simulink model "UAV_HIL"  (Simulink 8.0)
settings: Solver=ode3  StartTime=0.0  StopTime=inf  FixedStep=SampleTime  RelTol=1e-3
values from neighbouring files (symbols this model uses):
  SampleTime = 0.01    [setup.m]
undefined symbols (not defined in the file or in its folder): Serial_Port, Standard_Devices
undefined symbols (not defined in the file): AC
libraries: Actuator_Lib x2, rtwinlib x2, Environment_Lib x1, simulink x1, NonlinearModel_Lib x1, Sensors_Lib x1
CloseFcn:
  | rtwprivate ssgencode ModelCloseRequest Good_NL_model
settings Model: Creator=Paul  LastModifiedBy=brtaylor  SimulationMode=external  ExtModeTrigDuration=100000
settings DataIOCC: SignalLoggingSaveFormat=ModelDataLogs  TimeSaveName=time
settings OptimizationCC: InitFltsAndDblsToZero=on
settings DebuggingCC: ParameterPrecisionLossMsg=none  FcnCallInpInsideContextMsg=UseLocalSettings  StrictBusMsg=Warning
settings HardwareCC: ProdIntDivRoundTo=Zero  ProdEndianess=LittleEndian  ProdHWDeviceType=Generic->32-bit x86 compatible
settings SFSimCC: SimParseCustomCode=off
settings RTWCC: SystemTargetFile=rtwin.tlc  TemplateMakefile=rtwin.tmf  Description=Real-Time Windows Target  ProcessScript=rtwin_make_rtw_hook  RTWCompilerOptimization=On
settings CodeAppCC: MaxIdLength=95
settings RTWinTargetCC: TargetLibSuffix=_rtwin.lib  TargetPreCompLibLocation=C:\Program Files\MATLAB\R2012b\toolbox\rtw\targets\rtwin\lib\win64  CodeReplacementLibrary=ANSI_C  RTWinDir=C:/PROGRA~1/MATLAB/R2012b/toolbox/rtw/targets/rtwin  TargetArch=win64

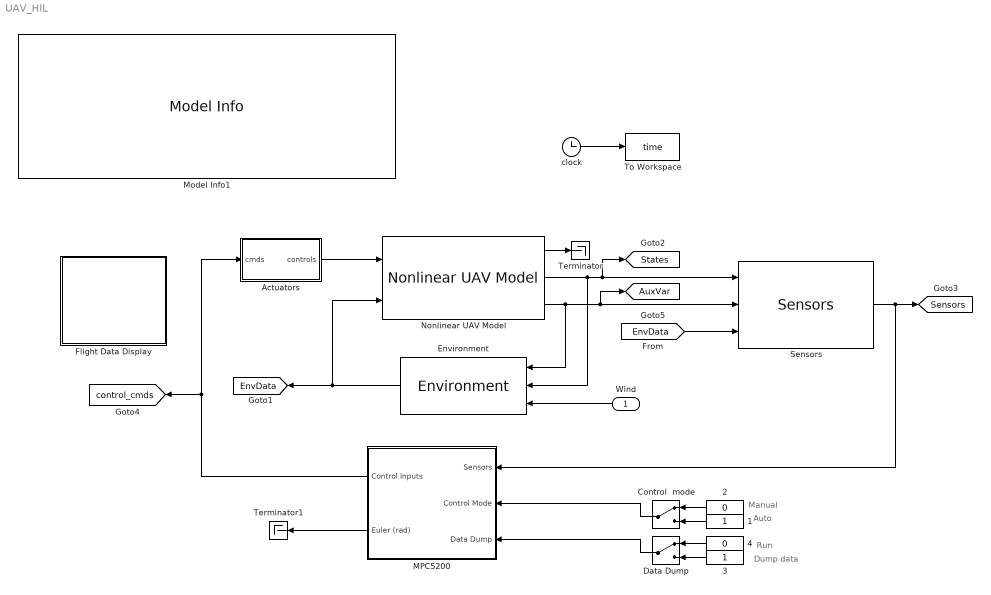
== system UAV_HIL ==
  note: Auto
  note: Run
  note: Dump data
  note: Manual
  Wind : Inport
  1 : Constant  OutDataTypeStr=uint8
  2 : Constant  Value=0  OutDataTypeStr=uint8
  3 : Constant  OutDataTypeStr=uint8
  4 : Constant  Value=0  OutDataTypeStr=uint8
  Actuators : Subsystem  BlockChoice=UltraStick  mask{aircraft=AC.aircraft}
      mask help: Set actuator models, either 'UltraStick120', 'UltraStick25e', or 'miniMUTT'
      mask init:
      | pathname = gcb;
      | 
      | switch lower(aircraft)
      |     case 'ultrastick120'
      |         set_param(pathname,'BlockChoice','UltraStick');
      |     case 'ultrastick25e'
      |         set_param(pathname,'BlockChoice','UltraStick');
      |     case 'minimutt'
      |         set_param(pathname,'BlockChoice','miniMUTT');
      | end
      settings: TemplateBlock=Actuator_Lib/Actuators  MemberBlocks=UltraStick,miniMUTT
  Control  mode : ManualSwitch
  Data Dump : ManualSwitch
  Environment : Environment_Lib/Environment
  Flight Data Display : Subsystem
      mask Display:
      | x = 0:.1:2*pi;
      | plot(x,sin(x)+rand(size(x))*.5)
  MPC5200 : Subsystem
  Model Info1 : simulink/Model-Wide Utilities/Model Info  InitialBlockCM=None  BlockCM=None  Frame=on  DisplayStringWithTags=|  HorizontalTextAlignment=Left  LeftAlignmentValue=0.02  SourceBlockDiagram=UAV_HIL  TagMaxNumber=20
      | MODEL INFORMATION
      | UMN UAV Hardware-in-the-Loop Simulation
      | 
      | University of Minnesota
      | Aerospace Engineering and Mechanics
      | Copyright 2011 Regents of the University of Minnesota. All rights reserved.
      | 
      | == SVN Info ==
      | Last modified by %<LastModifiedBy> on %<LastModificationDate>
  Nonlinear UAV Model : NonlinearModel_Lib/Nonlinear UAV Model
      link override Forces and Moments/Electric Propulsion Forces and Moments: BlockChoice=UltraStick
  Sensors : Sensors_Lib/Sensors
  Terminator : Terminator
  Terminator1 : Terminator
  To Workspace : ToWorkspace  VariableName=time  SampleTime=-1
  clock : Clock
  tag scope: AuxVar=global, EnvData=global, Sensors=global, States=global, control_cmds=global
  wires:
  2/1 -> Control  mode/1
  1/1 -> Control  mode/2
  Control  mode/1 -> MPC5200/2(Control Mode)
  4/1 -> Data Dump/1
  3/1 -> Data Dump/2
  Data Dump/1 -> MPC5200/3(Data Dump)
  Sensors/1 -> [Sensors], MPC5200/1(Sensors)
  Actuators/1(controls) -> Nonlinear UAV Model/1
  MPC5200/1(Control Inputs) -> Actuators/1(cmds), [control_cmds]
  clock/1 -> To Workspace/1
  Nonlinear UAV Model/2 -> Environment/2, [States], Sensors/1
  Nonlinear UAV Model/3 -> Environment/1, [AuxVar], Sensors/2
  Environment/1 -> [EnvData], Nonlinear UAV Model/2
  [EnvData] -> Sensors/3
  MPC5200/2(Euler (rad)) -> Terminator1/1
  Nonlinear UAV Model/1 -> Terminator/1
  Wind/1 -> Environment/3

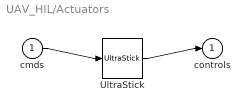
== system UAV_HIL/Actuators ==
  cmds : Inport
  UltraStick : Actuator_Lib/UltraStick
  controls : Outport
  wires:
  cmds/1 -> UltraStick/1
  UltraStick/1 -> controls/1

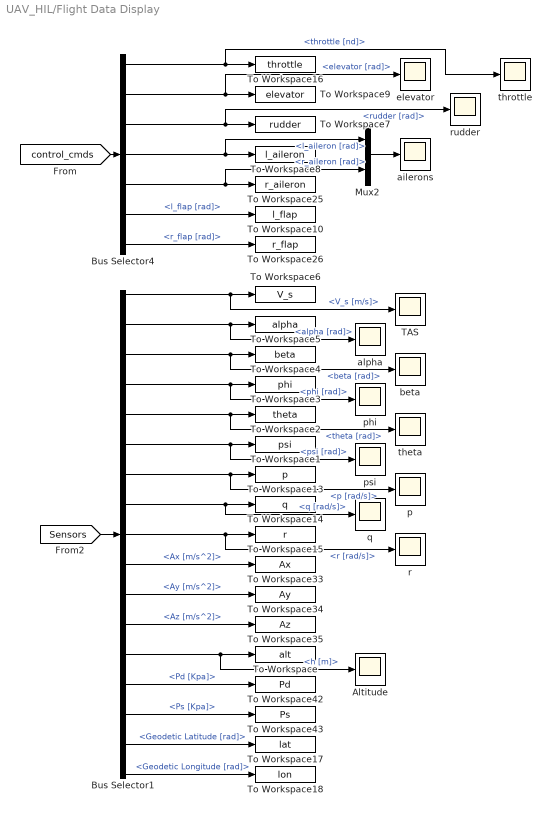
== system UAV_HIL/Flight Data Display ==
  Altitude : Scope
      settings: TimeRange=60  YMin=75  YMax=115  SaveName=ScopeData10
  Bus Selector1 : BusSelector  OutputSignals=V_s [m/s],alpha [rad],beta [rad],phi [rad],theta [rad],psi [rad],p [rad/s],q [rad/s],r [rad/s],Ax [m/s^2],Ay [m/s^2],Az [m/s^2],h [m],Pd [Kpa],Ps [Kpa],Geodetic Latitude [rad],Geodetic Longitude [rad]
  Bus Selector4 : BusSelector  OutputSignals=throttle [nd],elevator [rad],rudder [rad],l_aileron [rad],r_aileron [rad],l_flap [rad],r_flap [rad]
  Mux2 : Mux  Inputs=2
  TAS : Scope
      settings: TimeRange=45  YMin=14  YMax=19  SaveName=ScopeData3
  To Workspace : ToWorkspace  VariableName=alt  SampleTime=-1
  To Workspace1 : ToWorkspace  VariableName=psi  SampleTime=-1
  To Workspace10 : ToWorkspace  VariableName=l_flap  SampleTime=-1
  To Workspace13 : ToWorkspace  VariableName=p  SampleTime=-1
  To Workspace14 : ToWorkspace  VariableName=q  SampleTime=-1
  To Workspace15 : ToWorkspace  VariableName=r  SampleTime=-1
  To Workspace16 : ToWorkspace  VariableName=throttle  SampleTime=-1
  To Workspace17 : ToWorkspace  VariableName=lat  SampleTime=-1
  To Workspace18 : ToWorkspace  VariableName=lon  SampleTime=-1
  To Workspace2 : ToWorkspace  VariableName=theta  SampleTime=-1
  To Workspace25 : ToWorkspace  VariableName=r_aileron  SampleTime=-1
  To Workspace26 : ToWorkspace  VariableName=r_flap  SampleTime=-1
  To Workspace3 : ToWorkspace  VariableName=phi  SampleTime=-1
  To Workspace33 : ToWorkspace  VariableName=Ax  SampleTime=-1
  To Workspace34 : ToWorkspace  VariableName=Ay  SampleTime=-1
  To Workspace35 : ToWorkspace  VariableName=Az  SampleTime=-1
  To Workspace4 : ToWorkspace  VariableName=beta  SampleTime=-1
  To Workspace42 : ToWorkspace  VariableName=Pd  SampleTime=-1
  To Workspace43 : ToWorkspace  VariableName=Ps  SampleTime=-1
  To Workspace5 : ToWorkspace  VariableName=alpha  SampleTime=-1
  To Workspace6 : ToWorkspace  VariableName=V_s  SampleTime=-1
  To Workspace7 : ToWorkspace  VariableName=rudder  SampleTime=-1
  To Workspace8 : ToWorkspace  VariableName=l_aileron  SampleTime=-1
  To Workspace9 : ToWorkspace  VariableName=elevator  SampleTime=-1
  ailerons : Scope
      settings: TimeRange=20  YMin=-0.01  YMax=0.01  SaveName=ScopeData2
  alpha : Scope
      settings: TimeRange=25  YMin=0.035  YMax=0.08  SaveName=ScopeData7
  beta : Scope
      settings: TimeRange=25  YMin=-0.06  YMax=0.06  SaveName=ScopeData11
  elevator : Scope
      settings: TimeRange=45  YMin=-0.0961  YMax=-0.0961
  p : Scope
      settings: TimeRange=45  YMin=-1.675e-006  YMax=-1.4e-006  SaveName=ScopeData8
  phi : Scope
      settings: TimeRange=20  YMin=0.131875  YMax=0.132325  SaveName=ScopeData14
  psi : Scope
      settings: TimeRange=20  YMin=0  YMax=375  SaveName=ScopeData12
  q : Scope
      settings: TimeRange=45  YMin=-1e-009  YMax=1.5e-008  SaveName=ScopeData9
  r : Scope
      settings: TimeRange=45  YMin=-8  YMax=8
  rudder : Scope
      settings: TimeRange=45  YMin=0.0027  YMax=0.0027  SaveName=ScopeData4
  theta : Scope
      settings: TimeRange=20  YMin=0.0540123  YMax=0.0540123  SaveName=ScopeData13
  throttle : Scope
      settings: TimeRange=25  YMin=0.54169  YMax=0.59871  SaveName=ScopeData15
  wires:
  Bus Selector4/1 -> To Workspace16/1, throttle/1  "<throttle [nd]>"
  Bus Selector4/2 -> To Workspace9/1, elevator/1  "<elevator [rad]>"
  Bus Selector4/3 -> To Workspace7/1, rudder/1  "<rudder [rad]>"
  Bus Selector4/4 -> To Workspace8/1, Mux2/1  "<l_aileron [rad]>"
  Bus Selector4/5 -> To Workspace25/1, Mux2/2  "<r_aileron [rad]>"
  Bus Selector4/6 -> To Workspace10/1  "<l_flap [rad]>"
  Bus Selector4/7 -> To Workspace26/1  "<r_flap [rad]>"
  Mux2/1 -> ailerons/1
  [control_cmds] -> Bus Selector4/1
  [Sensors] -> Bus Selector1/1
  Bus Selector1/7 -> To Workspace13/1, p/1  "<p [rad/s]>"
  Bus Selector1/8 -> To Workspace14/1, q/1  "<q [rad/s]>"
  Bus Selector1/9 -> To Workspace15/1, r/1  "<r [rad/s]>"
  Bus Selector1/10 -> To Workspace33/1  "<Ax [m/s^2]>"
  Bus Selector1/11 -> To Workspace34/1  "<Ay [m/s^2]>"
  Bus Selector1/12 -> To Workspace35/1  "<Az [m/s^2]>"
  Bus Selector1/13 -> To Workspace/1, Altitude/1  "<h [m]>"
  Bus Selector1/14 -> To Workspace42/1  "<Pd [Kpa]>"
  Bus Selector1/15 -> To Workspace43/1  "<Ps [Kpa]>"
  Bus Selector1/16 -> To Workspace17/1  "<Geodetic Latitude [rad]>"
  Bus Selector1/17 -> To Workspace18/1  "<Geodetic Longitude [rad]>"
  Bus Selector1/6 -> To Workspace1/1, psi/1  "<psi [rad]>"
  Bus Selector1/1 -> To Workspace6/1, TAS/1  "<V_s [m/s]>"
  Bus Selector1/2 -> To Workspace5/1, alpha/1  "<alpha [rad]>"
  Bus Selector1/3 -> To Workspace4/1, beta/1  "<beta [rad]>"
  Bus Selector1/4 -> To Workspace3/1, phi/1  "<phi [rad]>"
  Bus Selector1/5 -> To Workspace2/1, theta/1  "<theta [rad]>"

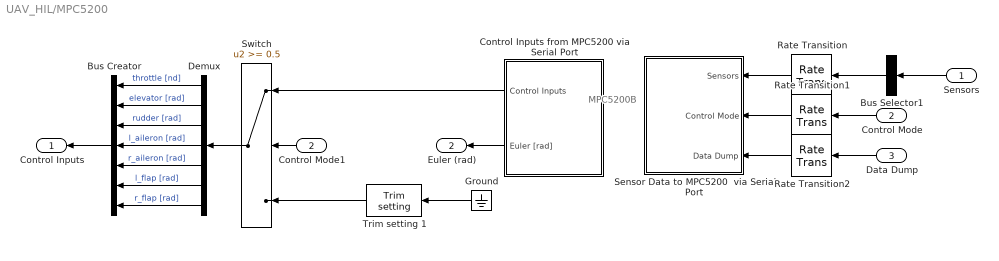
== system UAV_HIL/MPC5200 ==
  note: MPC5200B
  Sensors : Inport
  Control Mode : Inport  Port=2
  Data Dump : Inport  Port=3
  Bus Creator : BusCreator  Inputs=7
  Bus Selector1 : BusSelector  OutputSignals=p [rad/s],q [rad/s],r [rad/s],Ax [m/s^2],Ay [m/s^2],Az [m/s^2],Magnetic Field [nT],Geodetic Latitude [rad],Geodetic Longitude [rad],Altitude [m],Xdot [m/s],Ydot [m/s],Zdot [m/s],alpha [rad],beta [rad],Pd [Kpa],Ps [Kpa]  OutputAsBus=on
  Control Inputs from MPC5200 via Serial Port : Subsystem
  Control Mode1 : InportShadow  Port=2
  Demux : Demux  Outputs=7
  Ground : Ground
  Rate Transition : RateTransition  OutPortSampleTime=2*SampleTime
  Rate Transition1 : RateTransition  OutPortSampleTime=2*SampleTime
  Rate Transition2 : RateTransition  OutPortSampleTime=2*SampleTime
  Sensor Data to MPC5200  via Serial Port : Subsystem
  Switch : Switch  Threshold=0.5
  Trim setting 1 : Actuator_Lib/Trim setting 
  Control Inputs : Outport
  Euler (rad) : Outport  Port=2
  wires:
  Control Mode/1 -> Rate Transition1/1
  Sensors/1 -> Bus Selector1/1
  Data Dump/1 -> Rate Transition2/1
  Ground/1 -> Trim setting 1/1
  Control Mode1/1 -> Switch/2
  Demux/1 -> Bus Creator/1  "throttle [nd]"
  Demux/2 -> Bus Creator/2  "elevator [rad]"
  Demux/3 -> Bus Creator/3  "rudder [rad]"
  Demux/4 -> Bus Creator/4  "l_aileron [rad]"
  Demux/5 -> Bus Creator/5  "r_aileron [rad]"
  Demux/6 -> Bus Creator/6  "l_flap [rad]"
  Demux/7 -> Bus Creator/7  "r_flap [rad]"
  Bus Creator/1 -> Control Inputs/1
  Switch/1 -> Demux/1
  Control Inputs from MPC5200 via Serial Port/2(Euler [rad]) -> Euler (rad)/1
  Trim setting 1/1 -> Switch/3
  Control Inputs from MPC5200 via Serial Port/1(Control Inputs) -> Switch/1
  Rate Transition/1 -> Sensor Data to MPC5200  via Serial Port/1(Sensors)
  Rate Transition1/1 -> Sensor Data to MPC5200  via Serial Port/2(Control Mode)
  Rate Transition2/1 -> Sensor Data to MPC5200  via Serial Port/3(Data Dump)
  Bus Selector1/1 -> Rate Transition/1

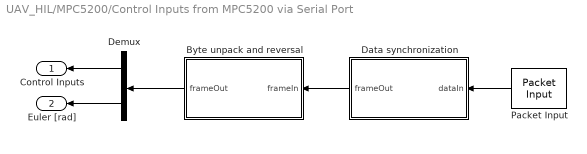
== system UAV_HIL/MPC5200/Control Inputs from MPC5200 via Serial Port ==
  Byte unpack and reversal : MATLAB Function  TreatAsAtomicUnit=on
  "Data synchronization " : MATLAB Function  TreatAsAtomicUnit=on
  Demux : Demux  Outputs=[7 3]
  Packet Input : rtwinlib/Packet Input  SampleTime=SampleTime  MaxMissedTicks=10  ShowMissedTicks=off  YieldWhenWaiting=off  DrvName=Standard_Devices/Serial_Port  DrvAddress=1  DrvOptions=[115200 8 0 0 0 0 0 0]  PacketSize=83  DataTypes='83*uint8'  ShowReady=off  ShowError=off  PacketID=1  ByteOrder=1  ShowTimestamp=off
      settings: AttributesFormatString=Standard Devices\nSerial Port [1h]
  Control Inputs : Outport
  Euler [rad] : Outport  Port=2
  wires:
  Packet Input/1 -> "Data synchronization "/1(dataIn)
  "Data synchronization "/1(frameOut) -> Byte unpack and reversal/1(frameIn)
  Demux/1 -> Control Inputs/1
  Demux/2 -> Euler [rad]/1
  Byte unpack and reversal/1(frameOut) -> Demux/1

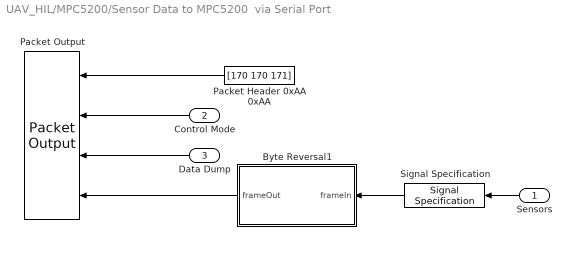
== system UAV_HIL/MPC5200/Sensor Data to MPC5200  via Serial Port ==
  Sensors : Inport
  Control Mode : Inport  Port=2
  Data Dump : Inport  Port=3
  Byte Reversal1 : MATLAB Function  TreatAsAtomicUnit=on
  Packet Header 0xAA 0xAA : Constant  Value=[170 170 171]  OutDataTypeStr=uint8
  Packet Output : rtwinlib/Packet Output  SampleTime=2*SampleTime  MaxMissedTicks=10  ShowMissedTicks=off  YieldWhenWaiting=off  DrvName=Standard_Devices/Serial_Port  DrvAddress=1  DrvOptions=[115200 8 0 0 0 0 0 0]  PacketSize=157  DataTypes={'3*uint8','uint8','uint8','19*double'}  ShowReady=off  ShowError=off  PacketID=1  ByteOrder=1  InitialValue=[]  FinalValue=[]
      settings: AttributesFormatString=Standard Devices\nSerial Port [1h]
  Signal Specification : SignalSpecification  OutDataTypeStr=double  Dimensions=19
  wires:
  Control Mode/1 -> Packet Output/2
  Signal Specification/1 -> Byte Reversal1/1(frameIn)
  Data Dump/1 -> Packet Output/3
  Sensors/1 -> Signal Specification/1
  Packet Header 0xAA 0xAA/1 -> Packet Output/1
  Byte Reversal1/1(frameOut) -> Packet Output/4

== matlab function MPC5200/Control Inputs from MPC5200 via Serial Port/Byte unpack and reversal ==
  data: frameIn input double; frameOut output double
function frameOut  = fcn(frameIn)
%#eml
%% Author: David Escobar Sanabria
%  Description: this function replaces byte unpack and byte reversal blocks
frameOut = zeros(10,1);
%frameIn2 = zeros(size(80,1));


for k=0:9 
    frameOut(k+1) = typecast((uint8([frameIn((k+1)*8:-1:k*8+1)])),'double');
end

== matlab function MPC5200/Control Inputs from MPC5200 via Serial Port/Data synchronization  ==
  data: dataIn input double; frameOut output double
function frameOut  = fcn(dataIn)
%#eml
%% Author: David Escobar Sanabria
%  Description: This function synchronizes data coming from the flight computer
%  computer. 
%  frameOut: Organized frame
%  frameIn: sequence of bytes not sync.
persistent frame; 
persistent lastFrame; 
persistent count; 
persistent countHeader; 
persistent countBuffer; 
persistent buffer; 

%% Size of byte array containing the data
sizePayload= 80;

%% Syze of the array read each time step
nBytes = 83 ;%size(dataIn,1); 


%%%%%%%%%%%%%%%%%%%%%%%%%%%%%%%%%%%%%%%%%%%%%%%%%%%%%%%
%% Initialization of presistent variables
if isempty(buffer)
    buffer=uint8(zeros(200,1));
end

if isempty(countBuffer)
    countBuffer=0;
end


if isempty(frame)
    frame=uint8(zeros(sizePayload,1));
end

if isempty(lastFrame)
    lastFrame=uint8(zeros(sizePayload,1));
end


if isempty(count)
    count=0;
end

if isempty(countHeader)
    countHeader=0;
end
%%%%%%%%%%%%%%%%%%%%%%%%%%%%%%%%%%%%%%%%%%%%%%%%%%%%%%%

%% Filling the buffer
buffer(countBuffer+1:countBuffer+nBytes) = dataIn;

bytesToRead = countBuffer+nBytes; 

%%%%%%%%%%%%%%%%%%%%%%%%%%%%%%%%%%%%%%%%%%%%%%%%%%%%%%%
%% Reading buffer

for k=1:bytesToRead    
    if(countHeader==3 && count<sizePayload)
        bytesLeft = sizePayload-count;
        frame(count+1:sizePayload) = buffer(k:k+bytesLeft-1);
        count = sizePayload;
        countBuffer = bytesToRead-bytesLeft ;
        buffer(1:countBuffer) = buffer(k+bytesLeft:bytesToRead);
        break;
        
    end
    
    if(countHeader==2 && buffer(k)==170)
        
        countHeader=3;
 
        if(bytesToRead-k > sizePayload)
            count =sizePayload;  
            frame(1:count) = buffer(k+1:k+sizePayload);  
            countBuffer =bytesToRead-k-sizePayload ; 
            buffer(1:countBuffer) = buffer(k+sizePayload+1:bytesToRead);
        else
            
            count =bytesToRead-k;
            if count > 0          
                frame(1:count) = buffer(k+1:bytesToRead);  
            end
            countBuffer = 0; 
            
        end
        
        break;
    end
    
    if(countHeader==1 && buffer(k)==171)
        countHeader=2;
    end
    
    if(countHeader==0 && buffer(k)==171)
        countHeader=1;
    end
        

end

if count==sizePayload 
     frameOut = frame;
     lastFrame = frame;
     frame=uint8(zeros(sizePayload,1));
     count=0;
     countHeader=0;
     
else % In case the buffer does not have an entire payload
    frameOut = lastFrame;
end

== matlab function MPC5200/Sensor Data to MPC5200 via Serial Port/Byte Reversal1 ==
  data: frameIn input double; frameOut output double
function frameOut  = fcn(frameIn)
%#eml
%% Author: David Escobar Sanabria
%  Description: this function replaces the byte reversal block
frameOut = zeros(19,1);

for k=1:19 
    %frameOut(k+1) = double([frameIn((k+1)*8:-1:k*8+1)]) ;
    
    vec = typecast(double(frameIn(k)),'uint8');
    frameOut(k) = typecast((uint8([vec(8:-1:1)])),'double');
    
end
